simulink model "req13B"  (R2019a)
settings: Solver=FixedStepAuto  StartTime=0.0  StopTime=100  RelTol=1e-3
settings Model: Creator=e40014285  LastModifiedBy=e40014285
settings ConfigComp: CovScope=ReferencedModels  CovHTMLOptions=-sRT=1 -sVT=0 -aTS=1 -bRG=1 -bTC=1 -hTR=0 -nFC=0 -nFD=1 -scm=1 -bcm=1 -xEv=0 -xEM=0  CovHtmlReporting=on  CovCumulativeReport=on  DVMaxProcessTime=6000  DVModelCoverageObjectives=EnhancedMCDC  DVTestSuiteOptimization=Auto  DVDetectOutOfBounds=on  DVReportPDFFormat=on  DVRebuildModelRepresentation=Always

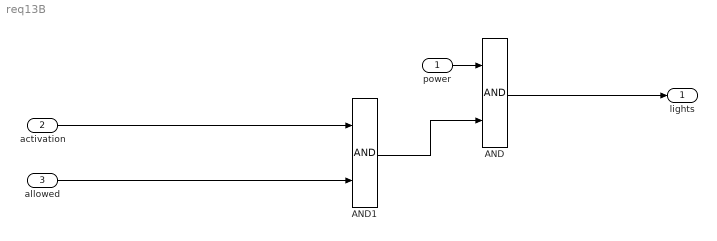
== system req13B ==
  power : Inport
  activation : Inport  Port=2
  allowed : Inport  Port=3
  AND : Logic  AllPortsSameDT=off  OutDataTypeStr=boolean
  AND1 : Logic  AllPortsSameDT=off  OutDataTypeStr=boolean
  lights : Outport
  wires:
  power/1 -> AND/1
  AND/1 -> lights/1
  AND1/1 -> AND/2
  activation/1 -> AND1/1
  allowed/1 -> AND1/2
